simulink model "chap02_61"  (R2013b)
settings: Solver=ode45  StartTime=0.0  StopTime=10.0  RelTol=1e-3
settings Model: Creator=Administrator  LastModifiedBy=sunzx.fnst

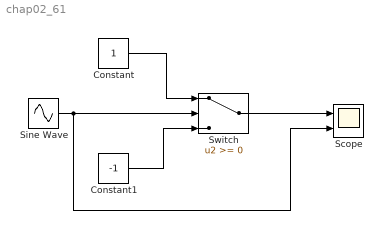
== system chap02_61 ==
  Constant : Constant
  Constant1 : Constant  Value=-1
  Scope : Scope  NumInputPorts=2
      settings: YMin=0.95~-1  YMax=1.05~1
  Sine Wave : Sin  SampleTime=0
  Switch : Switch
  wires:
  Constant/1 -> Switch/1
  Constant1/1 -> Switch/3
  Switch/1 -> Scope/1
  Sine Wave/1 -> Scope/2, Switch/2
